simulink model "etc_systemModeling"  (R2019b)
settings: Solver=FixedStepDiscrete  StartTime=0.0  StopTime=Inf  RelTol=1e-3  EnableMultiTasking=on
undefined symbols (not defined in the file): DiscIntNeverNeededParam, Down, GPTRIP1SEL, GPTRIP2SEL, TZ1, TZ2, Up
libraries: c2802xlib x5, dsparch4 x4, dspstat3 x4, simulink x3, c2837xDlib x1
settings Model: ExtModeTrigDuration=8  Creator=Nick  LastModifiedBy=Nick PC
settings OptimizationCC: DefaultUnderspecifiedDataType=single  EnhancedBackFolding=on  PassReuseOutputArgsAs=Individual arguments  MaxStackSize=1024  OptimizeBlockOrder=speed  DifferentSizesBufferReuse=on  OptimizationCustomize=off  DenormalBehavior=FlushToZero  EfficientTunableParamExpr=on
settings DebuggingCC: ParameterTunabilityLossMsg=error
settings HardwareCC: ProdBitPerChar=16  ProdBitPerInt=16  ProdBitPerPointer=32  ProdBitPerSizeT=32  ProdBitPerPtrDiffT=32  ProdLargestAtomicInteger=Integer  ProdLargestAtomicFloat=None  ProdWordSize=16  ProdLongLongMode=on  ProdHWDeviceType=Texas Instruments->C2000
settings SFSimCC: MATLABDynamicMemAlloc=off
settings RTWCC: SystemTargetFile=ert.tlc  HardwareBoard=TI Delfino F28377S LaunchPad  TLCOptions=-aInlineSetEventsForThisBaseRateFcn=TLC_FALSE -aSuppressMultiTaskScheduler=TLC_FALSE -aRateBasedStepFcn=1  TemplateMakefile=ert_default_tmf  GenerateReport=on  Toolchain=Texas Instruments Code Composer Studio (C2000)  IncludeHyperlinkInReport=on  LaunchReport=on  GenerateTraceInfo=on  GenerateTraceReport=on  GenerateTraceReportSl=on  GenerateTraceReportSf=on  GenerateTraceReportEml=on
settings CodeAppCC: ForceParamTrailComments=on  IgnoreCustomStorageClasses=off  OperatorAnnotations=on  SimulinkDataObjDesc=on  SFDataObjDesc=on  InsertBlockDesc=on
settings ERTTargetCC: CodeReplacementLibrary=TI C28x  ExtModeStaticAllocSize=10000

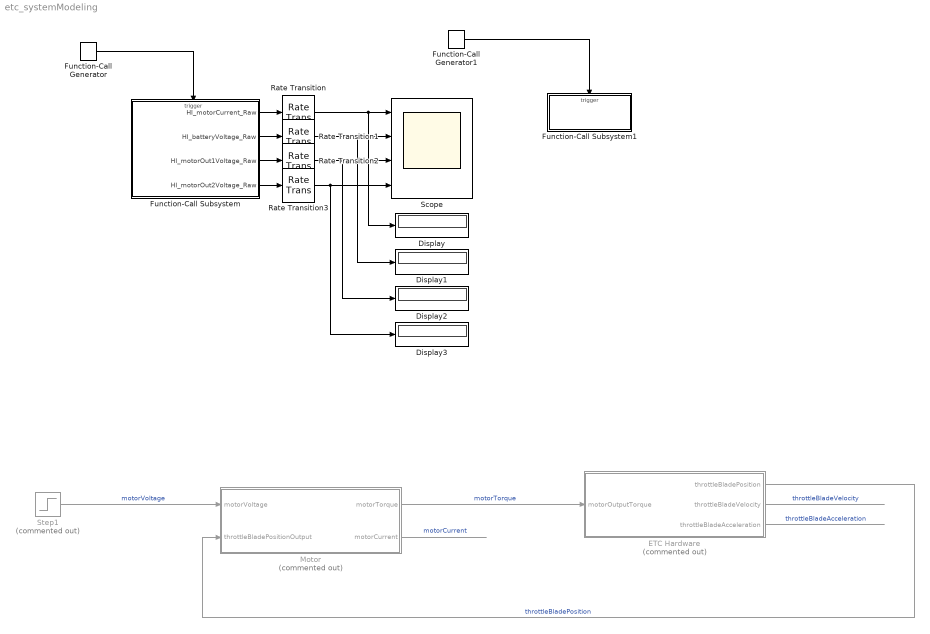
== system etc_systemModeling ==
  Display{,1..3} (4 alike) : Display
  ETC Hardware : Subsystem  Commented=on
  Function-Call Generator : simulink/Ports & Subsystems/Function-Call Generator  sample_time=.001  numberOfIterations=1
  Function-Call Generator1 : simulink/Ports & Subsystems/Function-Call Generator  sample_time=.01  numberOfIterations=1
  Function-Call Subsystem : Subsystem  TreatAsAtomicUnit=on
  Function-Call Subsystem1 : Subsystem  TreatAsAtomicUnit=on
  Motor : Subsystem  Commented=on
  Rate Transition{,1..3} (4 alike) : RateTransition
  Scope : Scope  NumInputPorts=4
  Step1 : Step  Commented=on  Time=0  After=4  SampleTime=0
  wires:
  Motor/1(motorTorque) -> ETC Hardware/1(motorOutputTorque)  "motorTorque"
  Motor/2(motorCurrent) -> ?  "motorCurrent"
  ETC Hardware/2(throttleBladeVelocity) -> ?  "throttleBladeVelocity"
  ETC Hardware/3(throttleBladeAcceleration) -> ?  "throttleBladeAcceleration"
  Step1/1 -> Motor/1(motorVoltage)  "motorVoltage"
  ETC Hardware/1(throttleBladePosition) -> Motor/2(throttleBladePositionOutput)  "throttleBladePosition"
  Function-Call Generator/1 -> Function-Call Subsystem/Trigger
  Function-Call Subsystem/4(HI_motorOut2Voltage_Raw) -> Rate Transition3/1
  Function-Call Subsystem/3(HI_motorOut1Voltage_Raw) -> Rate Transition2/1
  Function-Call Subsystem/2(HI_batteryVoltage_Raw) -> Rate Transition1/1
  Function-Call Subsystem/1(HI_motorCurrent_Raw) -> Rate Transition/1
  Function-Call Generator1/1 -> Function-Call Subsystem1/Trigger
  Rate Transition/1 -> Display/1, Scope/1
  Rate Transition1/1 -> Display1/1, Scope/2
  Rate Transition2/1 -> Display2/1, Scope/3
  Rate Transition3/1 -> Display3/1, Scope/4

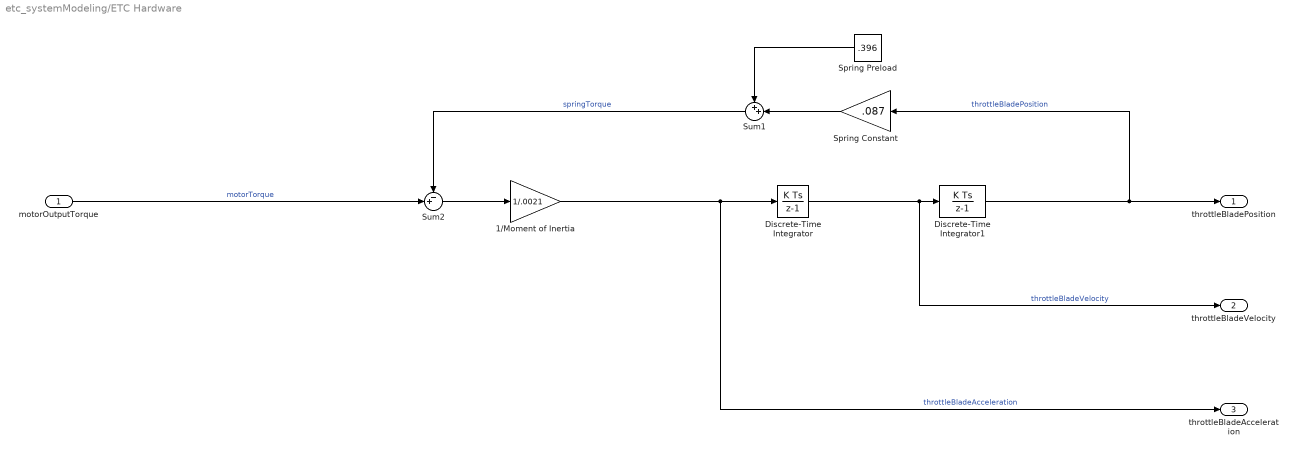
== system etc_systemModeling/ETC Hardware ==
  motorOutputTorque : Inport
  1/Moment of Inertia : Gain  Gain=1/.0021
  Discrete-Time Integrator : DiscreteIntegrator  SampleTime=-1  ICPrevOutput=DiscIntNeverNeededParam  ICPrevScaledInput=DiscIntNeverNeededParam
  Discrete-Time Integrator1 : DiscreteIntegrator  SampleTime=-1  LimitOutput=on  UpperSaturationLimit=1.5708  LowerSaturationLimit=0  ICPrevOutput=DiscIntNeverNeededParam  ICPrevScaledInput=DiscIntNeverNeededParam
  Spring Constant : Gain  Gain=.087
  Spring Preload : Constant  Value=.396
  Sum1 : Sum  Inputs=++|
  Sum2 : Sum  Inputs=-+|
  throttleBladePosition : Outport
  throttleBladeVelocity : Outport  Port=2
  throttleBladeAcceleration : Outport  Port=3
  wires:
  motorOutputTorque/1 -> Sum2/2  "motorTorque"
  Sum1/1 -> Sum2/1  "springTorque"
  1/Moment of Inertia/1 -> throttleBladeAcceleration/1, Discrete-Time Integrator/1  "throttleBladeAcceleration"
  Sum2/1 -> 1/Moment of Inertia/1
  Discrete-Time Integrator/1 -> throttleBladeVelocity/1, Discrete-Time Integrator1/1  "throttleBladeVelocity"
  Discrete-Time Integrator1/1 -> Spring Constant/1, throttleBladePosition/1  "throttleBladePosition"
  Spring Constant/1 -> Sum1/2
  Spring Preload/1 -> Sum1/1

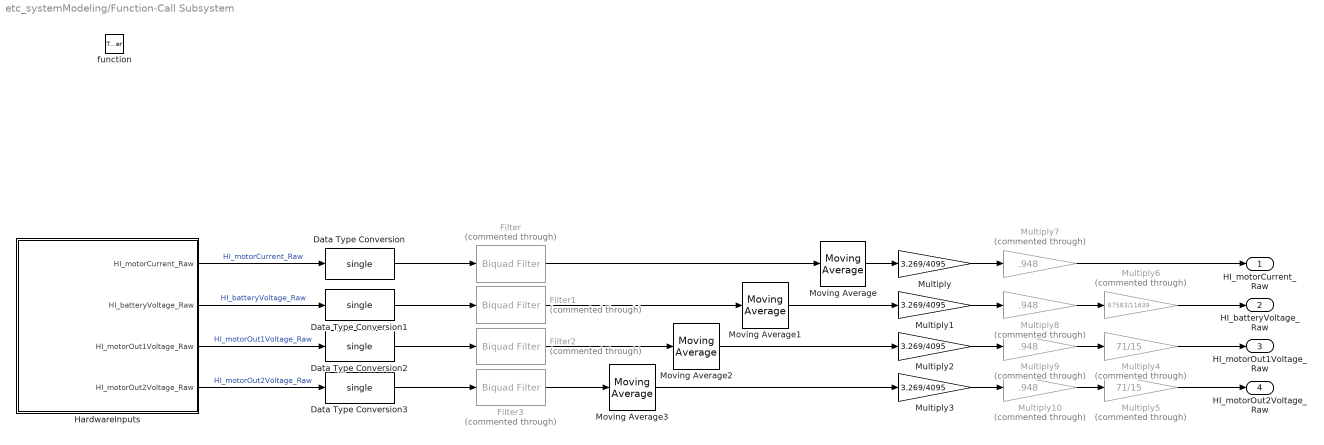
== system etc_systemModeling/Function-Call Subsystem ==
  function : TriggerPort  TriggerType=function-call  VariantControl=Variant
  Data Type Conversion{,1..3} (4 alike) : DataTypeConversion  OutDataTypeStr=single
  Filter{,1..3} (4 alike) : dsparch4/Biquad Filter  Tag=BlockMethodSubSystem  Commented=through  FilterSource=Dialog parameters  CoeffSource=Specify via dialog  FilterObject=BQF  IIRFiltStruct=Direct form II  BiQuadCoeffs=[1 1 0 1 -0.98751192990731429 0]  ScaleValues=[0.0062440350463428473;1]  IC=0  ICnum=0  ICden=0  a0Flag=Warning  optimizeScaleValues=on  ScaleValueMode=Specify via input port (g)  InputProcessing=Columns as channels (frame based)  roundingMode=Floor  overflowMode=off  scaleValueFracLength=14  denProdOutputFracLength=30  denAccumFracLength=30  secondMemoryFracLength=15
      settings: SourceProductName=DSP System Toolbox
  HardwareInputs : Subsystem
  Moving Average{,1..3} (4 alike) : dspstat3/Moving Average  Method=Sliding window  ForgettingFactorPort=off  SpecifyWindowLength=on  WindowLength=10  ForgettingFactor=0.9  SimulateUsing=Code generation
  Multiply{,1..3} (4 alike) : Gain  Gain=3.269/4095
  Multiply{7..10} (4 alike) : Gain  Commented=through  Gain=.948
  Multiply4 : Gain  Commented=through  Gain=71/15
  Multiply5 : Gain  Commented=through  Gain=71/15
  Multiply6 : Gain  Commented=through  Gain=67583/11639
  HI_motorCurrent_Raw : Outport
  HI_batteryVoltage_Raw : Outport  Port=2
  HI_motorOut1Voltage_Raw : Outport  Port=3
  HI_motorOut2Voltage_Raw : Outport  Port=4
  wires:
  HardwareInputs/1(HI_motorCurrent_Raw) -> Data Type Conversion/1  "HI_motorCurrent_Raw"
  HardwareInputs/2(HI_batteryVoltage_Raw) -> Data Type Conversion1/1  "HI_batteryVoltage_Raw"
  HardwareInputs/3(HI_motorOut1Voltage_Raw) -> Data Type Conversion2/1  "HI_motorOut1Voltage_Raw"
  HardwareInputs/4(HI_motorOut2Voltage_Raw) -> Data Type Conversion3/1  "HI_motorOut2Voltage_Raw"
  Moving Average/1 -> Multiply/1
  Moving Average1/1 -> Multiply1/1
  Moving Average2/1 -> Multiply2/1
  Moving Average3/1 -> Multiply3/1
  Data Type Conversion/1 -> Filter/1
  Data Type Conversion1/1 -> Filter1/1
  Data Type Conversion2/1 -> Filter2/1
  Data Type Conversion3/1 -> Filter3/1
  Filter/1 -> Moving Average/1
  Filter1/1 -> Moving Average1/1
  Filter2/1 -> Moving Average2/1
  Filter3/1 -> Moving Average3/1
  Multiply/1 -> Multiply7/1
  Multiply1/1 -> Multiply8/1
  Multiply2/1 -> Multiply9/1
  Multiply3/1 -> Multiply10/1
  Multiply4/1 -> HI_motorOut1Voltage_Raw/1
  Multiply5/1 -> HI_motorOut2Voltage_Raw/1
  Multiply6/1 -> HI_batteryVoltage_Raw/1
  Multiply7/1 -> HI_motorCurrent_Raw/1
  Multiply8/1 -> Multiply6/1
  Multiply9/1 -> Multiply4/1
  Multiply10/1 -> Multiply5/1

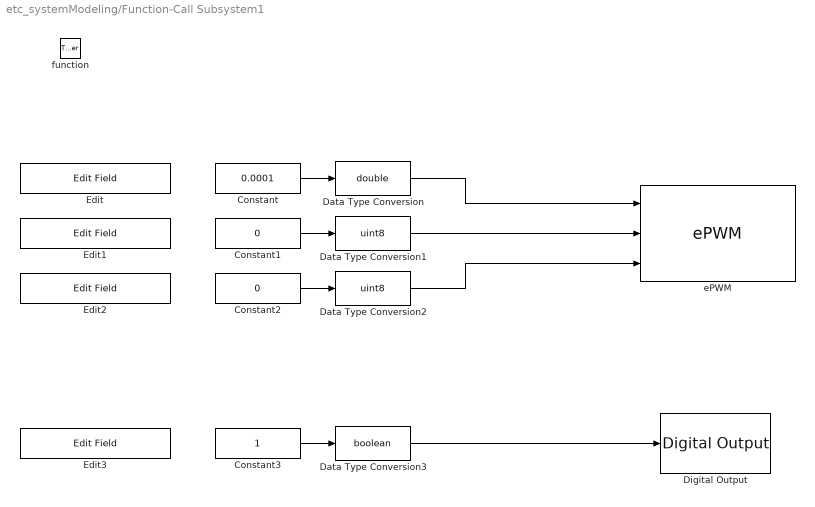
== system etc_systemModeling/Function-Call Subsystem1 ==
  function : TriggerPort  TriggerType=function-call  VariantControl=Variant
  Constant : Constant  Value=0.0001
  Constant1 : Constant  Value=0
  Constant2 : Constant  Value=0
  Constant3 : Constant
  Data Type Conversion : DataTypeConversion  OutDataTypeStr=double
  Data Type Conversion1 : DataTypeConversion  OutDataTypeStr=uint8
  Data Type Conversion2 : DataTypeConversion  OutDataTypeStr=uint8
  Data Type Conversion3 : DataTypeConversion  OutDataTypeStr=boolean
  Digital Output : c2837xDlib/Digital Output  GPIO_Number=GPIO40~GPIO47  GPIO_Bit0=off  GPIO_BIT0_Toggle=off  GPIO_Bit1=on  GPIO_BIT1_Toggle=off  GPIO_Bit2=off  GPIO_BIT2_Toggle=off  GPIO_Bit3=off  GPIO_BIT3_Toggle=off  GPIO_Bit4=off  GPIO_BIT4_Toggle=off  GPIO_Bit5=off  GPIO_BIT5_Toggle=off  GPIO_Bit6=off  GPIO_BIT6_Toggle=off  GPIO_Bit7=off  GPIO_BIT7_Toggle=off
      settings: SourceProductName=Embedded Coder Support Package for Texas Instruments C2000 Processors  SourceProductBaseCode=TIC2000
  Edit{,1..3} (4 alike) : EditField  LabelPosition=Hide  ShowInitialText=on  Alignment=Center
  ePWM : c2802xlib/ePWM  useModule=ePWM8  ePWMxLINKTBPRD=Not Linked  periodUnits=Seconds  timerSource=Input port  timerPeriod_clk=64000  timerPeriod_sec=0.0001  tbshadow=Counter equals to zero  countingMode=Up-Down  phaseActiveEnable=Disable  phaseDirection=Count down after sync  phaseActive=0  synchronizationEnable=off  dcaevt1Sync=off  dcbevt1Sync=off  synchronizationOption=Disable  clockPrescale=1  HSclockPrescale=1  enswap=off  ePWMxAStatus=on  ePWMxAactionLogic1=Set  ePWMxAactionLogic2=Clear  ePWMxAactionLogic3=Clear  ePWMxAactionLogic4=Set  ePWMxAactionLogic5=Do nothing  ePWMxAactionLogic6=Do nothing  ePWMxALoadMode=Load on counter equals to zero (CTR=Zero)  ePWMxACSFenable=off  ePWMxACSFvalue=Forcing disable  ePWMxASFreload=Zero  ePWMxBStatus=on  ePWMxBactionLogic1=Set  ePWMxBactionLogic2=Clear  ePWMxBactionLogic3=Do nothing  ePWMxBactionLogic4=Do nothing  ePWMxBactionLogic5=Clear  ePWMxBactionLogic6=Set  ePWMxBLoadMode=Load on counter equals to zero (CTR=Zero)  ePWMxBCSFenable=off  ePWMxBCSFvalue=Forcing disable  ePWMxBSFreload=Zero  ePWNxBOutWay=off  ePWMxLINKCMPA=Not Linked  CMPAUnits=Percentages  CMPASource=Input port  CMPAValue_per=0  CMPAValue_clk=32000  enCMPAshadow=Counter equals to zero  ePWMxLINKCMPB=Not Linked  CMPBUnits=Percentages  CMPBSource=Input port  CMPBValue_per=0  CMPBValue_clk=32000  enCMPBshadow=Counter equals to zero  ePWMxLINKCMPC=Not Linked  CMPCUnits=Clock cycles  CMPCSource=Specify via dialog  CMPCValue_per=50  CMPCValue_clk=32000  enCMPCshadow=Counter equals to zero  ePWMxLINKCMPD=Not Linked  CMPDUnits=Clock cycles  CMPDSource=Specify via dialog  CMPDValue_per=50  CMPDValue_clk=32000  enCMPDshadow=Counter equals to zero  enableDBePWMxA=off  enableDBePWMxB=off  enhalfcycle=off  DBpolarity=Active high (AH)  DBedgeDelay=Positive  DBSource_ePWMxA=ePWMxA  DBSource_ePWMxB=ePWMxA  DBperiodSource=Specify via dialog  REDperiod=0  FEDperiod=0  adcstartModuleA=off  adcrequestEventA=First event  adcstartEventA=Digital Compare Module A Event 1 start of conversion (DCAEVT1.soc)  adcstartEventA_type2=Digital Compare Module A Event 1 start of conversion (DCAEVT1.soc)  adcstartModuleB=off  adcrequestEventB=First event  adcstartEventB=Counter equals to zero (CTR=Zero)  adcstartEventB_type2=Counter equals to zero (CTR=Zero)  intEn=off  intPrd=First event  intSel=Counter equals to zero (CTR=Zero)  intSel_type2=Counter equals to zero (CTR=Zero)  hrpe=off  enHRPWM=off  HRPWM_LoadMode=Counter equals to period (CTR=PRD)  HRPWM_CTLMode=Duty or Period control mode  HRPWM_EDGMode=Both edge  hrpeb=off  enHRPWMB=off  HRPWM_LoadModeB=Counter equals to zero (CTR=ZERO)  HRPWM_CTLModeB=Duty or Period control mode  HRPWM_EDGModeB=Both edge  enSFO=on  enautoconv=on  chopperEnable=off  chopperFrequency=1  chopperFirstwidth=1  chopperDuty=12.5%  tripZonesource=Specify via dialog  tzselOSHT1=off  tzselOSHT2=off  tzselOSHT3=off  tzselOSHDCAEV1=off  tzselOSHDCBEV1=off  tzselCBC1=off  tzselCBC2=off  tzselCBC3=off  tzselCBCDCAEV2=off  tzselCBCDCBEV2=off  tzselOSHT4=off  tzselOSHT5=off  tzselOSHT6=off  tzselCBC4=off  tzselCBC5=off  tzselCBC6=off  enTzOstIntr=off  enTzCbcIntr=off  enTzDCAEVT1Intr=off  enTzDCAEVT2Intr=off  enTzDCBEVT1Intr=off  enTzDCBEVT2Intr=off  ePWMxAforced=No action  ePWMxBforced=No action  DCAEVT1forced=No action  DCBEVT1forced=No action  DCAEVT2forced=No action  DCBEVT2forced=No action  dcah=Trip Zone 1 input (TZ1)  dcal=Trip Zone 2 input (TZ2)  dcbh=Trip Zone 1 input (TZ1)  dcbl=Trip Zone 2 input (TZ2)  dcah_type2=GPTRIP1SEL/(TZ1)  dcal_type2=GPTRIP2SEL/(TZ2)  dcbh_type2=GPTRIP1SEL/(TZ1)  dcbl_type2=GPTRIP2SEL/(TZ2)  gendcaevt1=Event disabled  gendcaevt2=Event disabled  gendcbevt1=Event disabled  gendcbevt2=Event disabled  dcaevt1src=DCAEVT1 with sync  dcaevt2src=DCAEVT2 with sync  dcbevt1src=DCBEVT1 with sync  dcbevt2src=DCBEVT2 with sync  pulsesel=Counter equals to zero (CTR=Zero)  blankinv=off  blankoffset=0  blankwidth=0  evsrcsel=Filtered version of DCAEVT1 (DCAEVT1FILT)  encape=off  PwmType=C2000_Type4
      settings: SourceProductName=Embedded Coder Support Package for Texas Instruments C2000 Processors
  wires:
  Constant1/1 -> Data Type Conversion1/1
  Constant/1 -> Data Type Conversion/1
  Constant2/1 -> Data Type Conversion2/1
  Data Type Conversion/1 -> ePWM/1
  Data Type Conversion1/1 -> ePWM/2
  Data Type Conversion2/1 -> ePWM/3
  Constant3/1 -> Data Type Conversion3/1
  Data Type Conversion3/1 -> Digital Output/1

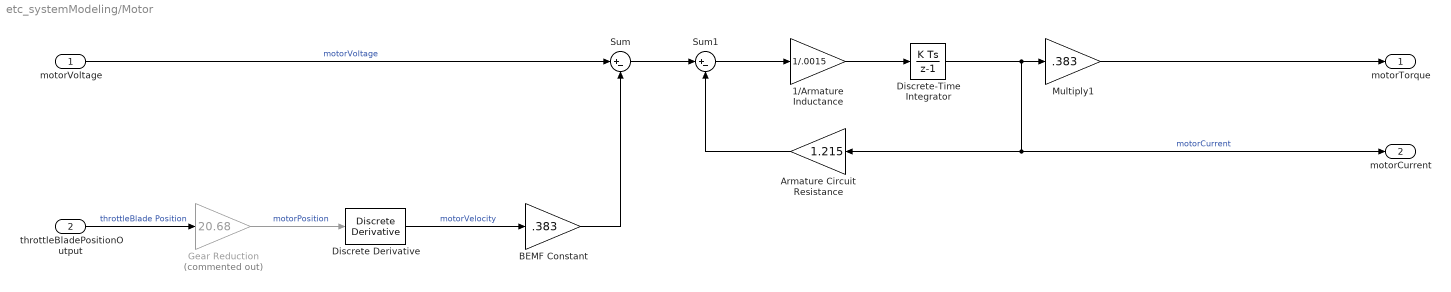
== system etc_systemModeling/Motor ==
  motorVoltage : Inport
  throttleBladePositionOutput : Inport  Port=2
  1/Armature Inductance : Gain  Gain=1/.0015
  Armature Circuit Resistance : Gain  Gain=1.215
  BEMF Constant : Gain  Gain=.383
  Discrete Derivative : simulink/Discrete/Discrete Derivative  gainval=1.0  ICPrevScaledInput=0.0  OutMin=[]  OutMax=[]  OutDataType=fixdt(1, 16)  OutScaling=2^-10  DoSatur=off
  Discrete-Time Integrator : DiscreteIntegrator  SampleTime=-1  ICPrevOutput=DiscIntNeverNeededParam  ICPrevScaledInput=DiscIntNeverNeededParam
  Gear Reduction : Gain  Commented=on  Gain=20.68
  Multiply1 : Gain  Gain=.383
  Sum : Sum  Inputs=|+-
  Sum1 : Sum  Inputs=|+-
  motorTorque : Outport
  motorCurrent : Outport  Port=2
  wires:
  Discrete-Time Integrator/1 -> Armature Circuit Resistance/1, motorCurrent/1, Multiply1/1  "motorCurrent"
  Multiply1/1 -> motorTorque/1
  motorVoltage/1 -> Sum/1  "motorVoltage"
  Armature Circuit Resistance/1 -> Sum1/2
  Sum1/1 -> 1/Armature Inductance/1
  1/Armature Inductance/1 -> Discrete-Time Integrator/1
  Sum/1 -> Sum1/1
  BEMF Constant/1 -> Sum/2
  throttleBladePositionOutput/1 -> Gear Reduction/1  "throttleBlade Position"
  Gear Reduction/1 -> Discrete Derivative/1  "motorPosition"
  Discrete Derivative/1 -> BEMF Constant/1  "motorVelocity"

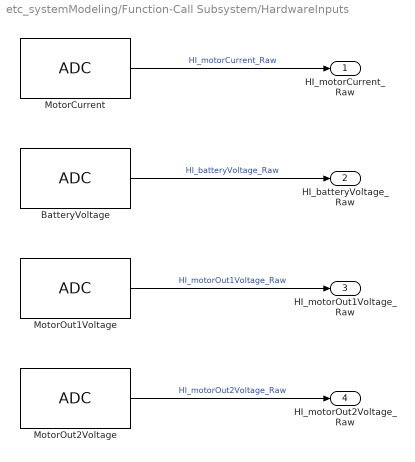
== system etc_systemModeling/Function-Call Subsystem/HardwareInputs ==
  BatteryVoltage : c2802xlib/ADC  blkParamProc=C2000_Type4  ADCModule=B  samplingMode=Single sample mode  ADCResolution=12-bit (Single-ended input)  useSOC1=SOC1  useSOC2=SOC0_SOC1  SOCAcquisitionWindow=15  SOCTriggerSource=Software  SOCInterruptTrigger=No ADCINT  Ts=-1  dType=uint16  postInterrupt=off  interruptSel=ADCINT1  ADCINTContinuous=on  endma=off  chdma=1  conv1=ADCINA0  conv2=ADCINA0 and ADCINB0  conv1_Type4=ADCIN1  conv2_Type4=ADCIN0 and ADCIN1
      settings: SourceProductName=Embedded Coder Support Package for Texas Instruments C2000 Processors
  MotorCurrent : c2802xlib/ADC  blkParamProc=C2000_Type4  ADCModule=B  samplingMode=Single sample mode  ADCResolution=12-bit (Single-ended input)  useSOC1=SOC0  useSOC2=SOC0_SOC1  SOCAcquisitionWindow=15  SOCTriggerSource=Software  SOCInterruptTrigger=No ADCINT  Ts=-1  dType=uint16  postInterrupt=off  interruptSel=ADCINT1  ADCINTContinuous=on  endma=off  chdma=1  conv1=ADCINA0  conv2=ADCINA0 and ADCINB0  conv1_Type4=ADCIN2  conv2_Type4=ADCIN0 and ADCIN1
      settings: SourceProductName=Embedded Coder Support Package for Texas Instruments C2000 Processors
  MotorOut1Voltage : c2802xlib/ADC  blkParamProc=C2000_Type4  ADCModule=B  samplingMode=Single sample mode  ADCResolution=12-bit (Single-ended input)  useSOC1=SOC2  useSOC2=SOC0_SOC1  SOCAcquisitionWindow=15  SOCTriggerSource=Software  SOCInterruptTrigger=No ADCINT  Ts=-1  dType=uint16  postInterrupt=off  interruptSel=ADCINT1  ADCINTContinuous=on  endma=off  chdma=1  conv1=ADCINA0  conv2=ADCINA0 and ADCINB0  conv1_Type4=ADCIN4  conv2_Type4=ADCIN0 and ADCIN1
      settings: SourceProductName=Embedded Coder Support Package for Texas Instruments C2000 Processors
  MotorOut2Voltage : c2802xlib/ADC  blkParamProc=C2000_Type4  ADCModule=B  samplingMode=Single sample mode  ADCResolution=12-bit (Single-ended input)  useSOC1=SOC3  useSOC2=SOC0_SOC1  SOCAcquisitionWindow=15  SOCTriggerSource=Software  SOCInterruptTrigger=No ADCINT  Ts=-1  dType=uint16  postInterrupt=off  interruptSel=ADCINT1  ADCINTContinuous=on  endma=off  chdma=1  conv1=ADCINA0  conv2=ADCINA0 and ADCINB0  conv1_Type4=ADCIN14  conv2_Type4=ADCIN0 and ADCIN1
      settings: SourceProductName=Embedded Coder Support Package for Texas Instruments C2000 Processors
  HI_motorCurrent_Raw : Outport
  HI_batteryVoltage_Raw : Outport  Port=2
  HI_motorOut1Voltage_Raw : Outport  Port=3
  HI_motorOut2Voltage_Raw : Outport  Port=4
  wires:
  MotorCurrent/1 -> HI_motorCurrent_Raw/1  "HI_motorCurrent_Raw"
  BatteryVoltage/1 -> HI_batteryVoltage_Raw/1  "HI_batteryVoltage_Raw"
  MotorOut1Voltage/1 -> HI_motorOut1Voltage_Raw/1  "HI_motorOut1Voltage_Raw"
  MotorOut2Voltage/1 -> HI_motorOut2Voltage_Raw/1  "HI_motorOut2Voltage_Raw"
